simulink model "RollYawMissile_sim"  (R2016a)
settings: Solver=ode15s  StartTime=0.0  StopTime=10  MaxStep=0.1
libraries: cstblocks x9
settings Model: Creator=fbianchi  LastModifiedBy=ferna
settings SolverCC: SolverResetMethod=Robust
settings DataIOCC: LimitDataPoints=on  SaveFormat=Array  SignalLoggingSaveFormat=ModelDataLogs
settings OptimizationCC: ExpressionDepthLimit=2147483647  InitFltsAndDblsToZero=on
settings DebuggingCC: AlgebraicLoopMsg=none  SaveWithParameterizedLinksMsg=none  UnderspecifiedInitializationDetection=Classic  MergeDetectMultiDrivingBlocksExec=none  SignalResolutionControl=TryResolveAllWithWarning  SolverPrmCheckMsg=warning  MultiTaskDSMMsg=warning  MultiTaskCondExecSysMsg=none  FcnCallInpInsideContextMsg=UseLocalSettings  StateNameClashWarn=warning
settings HardwareCC: ProdBitPerPointer=32  ProdLargestAtomicFloat=None  ProdIntDivRoundTo=Undefined  ProdEndianess=Unspecified  ProdWordSize=32  ProdHWDeviceType=32-bit Generic
settings ModelReferenceCC: PropagateSignalLabelsOutOfModel=off
settings GRTTargetCC: TargetFcnLib=ansi_tfl_tmw.mat  CombineOutputUpdateFcns=off  GRTInterface=on
settings ConfigComp: CovModelRefEnable=Off

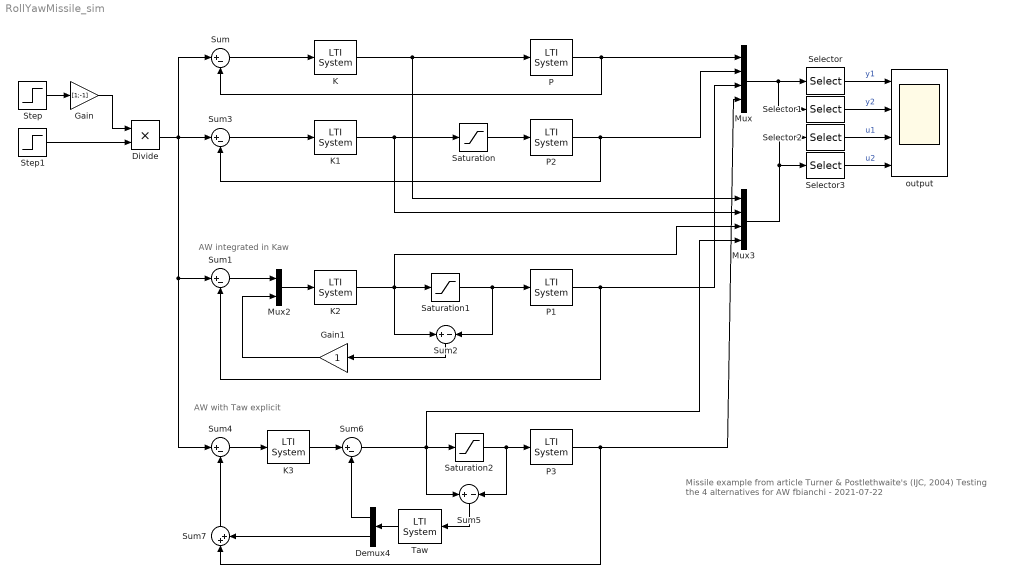
== system RollYawMissile_sim ==
  note: AW integrated in Kaw
  note: AW with Taw explicit
  note: Missile example from article Turner & Postlethwaite's
      | (IJC, 2004)
      |
      | Testing the 4 alternatives for AW
      |
      | fbianchi - 2021-07-22
  Demux4 : Demux  Outputs=[2 2]
  Divide : Product  Inputs=**
  Gain : Gain  Gain=[1;-1]
  Gain1 : Gain
  K : cstblocks/LTI System  sys=C  IC=0
  K1 : cstblocks/LTI System  sys=C  IC=0
  K2 : cstblocks/LTI System  sys=Kaw  IC=0
  K3 : cstblocks/LTI System  sys=C  IC=0
  Mux : Mux  Inputs=[2 2 2 2]
  Mux2 : Mux  Inputs=2
  Mux3 : Mux  Inputs=[2 2 2 2]
  P{,1..3} (4 alike) : cstblocks/LTI System  sys=P  IC=0
  Saturation : Saturate  UpperLimit=8  LowerLimit=-8
  Saturation1 : Saturate  UpperLimit=8  LowerLimit=-8
  Saturation2 : Saturate  UpperLimit=8  LowerLimit=-8
  Selector : Selector  InputPortWidth=8  IndexOptions=Index vector (dialog)  Indices=[1 3 5 7]  OutputSizes=1
  Selector1 : Selector  InputPortWidth=8  IndexOptions=Index vector (dialog)  Indices=[2 4 6 8]  OutputSizes=1
  Selector2 : Selector  InputPortWidth=8  IndexOptions=Index vector (dialog)  Indices=[1 3 5 7]  OutputSizes=1
  Selector3 : Selector  InputPortWidth=8  IndexOptions=Index vector (dialog)  Indices=[2 4 6 8]  OutputSizes=1
  Step : Step  After=4.2  SampleTime=0
  Step1 : Step  Time=5  Before=1  After=0  SampleTime=0
  Sum{,1,3..4,6} (5 alike) : Sum  Inputs=|+-
  Sum2 : Sum  Inputs=+-
  Sum5 : Sum  Inputs=+-
  Sum7 : Sum  Inputs=|++
  Taw : cstblocks/LTI System  sys=Taw  IC=0
  output : Scope  NumInputPorts=4
  wires:
  Sum/1 -> K/1
  P/1 -> Mux/1, Sum/2
  K/1 -> P/1, Mux3/1
  Step/1 -> Gain/1
  P1/1 -> Mux/3, Sum1/2
  P2/1 -> Sum3/2, Mux/2
  K1/1 -> Saturation/1, Mux3/2
  Saturation/1 -> P2/1
  Sum1/1 -> Mux2/1
  Mux2/1 -> K2/1
  K2/1 -> Mux3/3, Saturation1/1, Sum2/1
  Gain/1 -> Divide/1
  Step1/1 -> Divide/2
  Sum3/1 -> K1/1
  Saturation1/1 -> P1/1, Sum2/2
  Sum2/1 -> Gain1/1
  P3/1 -> Sum7/1, Mux/4
  Sum4/1 -> K3/1
  Saturation2/1 -> Sum5/2, P3/1
  K3/1 -> Sum6/1
  Sum6/1 -> Saturation2/1, Mux3/4, Sum5/1
  Taw/1 -> Demux4/1
  Sum7/1 -> Sum4/2
  Mux3/1 -> Selector3/1, Selector2/1
  Divide/1 -> Sum4/1, Sum1/1, Sum/1, Sum3/1
  Gain1/1 -> Mux2/2
  Mux/1 -> Selector/1, Selector1/1
  Selector/1 -> output/1  "y1"
  Selector1/1 -> output/2  "y2"
  Selector2/1 -> output/3  "u1"
  Selector3/1 -> output/4  "u2"
  Demux4/1 -> Sum6/2
  Demux4/2 -> Sum7/2
  Sum5/1 -> Taw/1
